simulink model "Q1"  (R2020b)
settings: Solver=VariableStepAuto  StartTime=0.0  StopTime=10.0  RelTol=1e-3
undefined symbols (not defined in the file): b, k1, k12
settings Model: Creator=HP  LastModifiedBy=HP

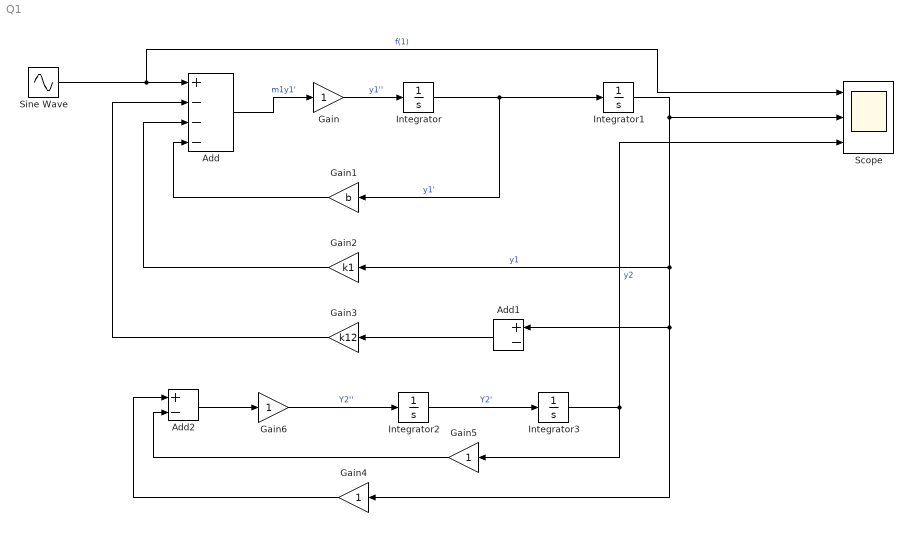
== system Q1 ==
  Add : Sum  Inputs=+---
  Add1 : Sum  Inputs=+-
  Add2 : Sum  Inputs=+-
  Gain{,4..6} (4 alike) : Gain
  Gain1 : Gain  Gain=b
  Gain2 : Gain  Gain=k1
  Gain3 : Gain  Gain=k12
  Integrator{,1..3} (4 alike) : Integrator
  Scope : Scope  NumInputPorts=3
  Sine Wave : Sin  SampleTime=0
  wires:
  Add/1 -> Gain/1  "m1y1'"
  Gain/1 -> Integrator/1  "y1''"
  Integrator/1 -> Gain1/1, Integrator1/1  "y1'"
  Gain1/1 -> Add/4
  Gain2/1 -> Add/3
  Integrator1/1 -> Scope/2, Gain4/1, Add1/1, Gain2/1  "y1"
  Gain3/1 -> Add/2
  Add1/1 -> Gain3/1
  Add2/1 -> Gain6/1
  Gain6/1 -> Integrator2/1  "Y2''"
  Integrator2/1 -> Integrator3/1  "Y2'"
  Gain5/1 -> Add2/2
  Gain4/1 -> Add2/1
  Integrator3/1 -> Scope/3, Gain5/1  "y2"
  Sine Wave/1 -> Scope/1, Add/1  "f(1)"
